simulink library "rlsGradientEst_cl"  (R2018b)
settings: Solver=VariableStepAuto  StartTime=0.0  StopTime=10.0  RelTol=1e-3
undefined symbols (not defined in the file): AdaptationParameter, initBasisParams
libraries: ctrlSharedLib x1
settings Model: Creator=mcobb  LastModifiedBy=mcobb

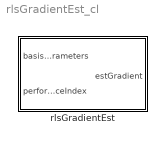
== system rlsGradientEst_cl ==
  rlsGradientEst : Subsystem  mask{InitialParameterData=ones([2*numel(initBasisParams)+1 1]), AdaptationParameter=AdaptationParameter, Ts=1}
      mask prompts: InitialParameterData "Controllib:blocks:recursiveEstimationMaskInitialParameterValues"; AdaptationParameter "Controllib:blocks:recursiveEstimationMaskAdaptationParameterFF"; Ts "Sample Time"
      mask TypeOptions InitialParameterData: Recursive Least Squares Estimator/InitialParameterData
      mask TypeOptions AdaptationParameter: Recursive Least Squares Estimator/AdaptationParameter
      mask DialogControl InitialParameterData Prompt: Initial Parameter Values:
      mask DialogControl AdaptationParameter Prompt: Forgetting Factor:

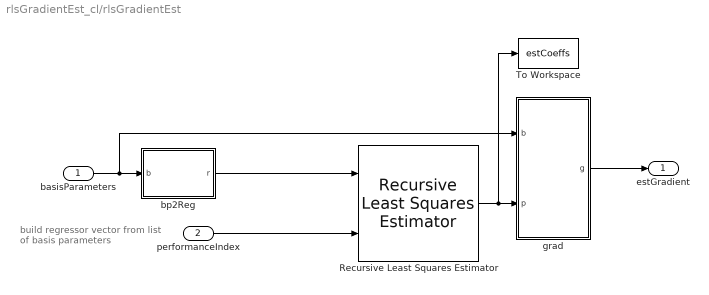
== system rlsGradientEst_cl/rlsGradientEst ==
  note: build regressor vector from
      | list of basis parameters
  basisParameters : Inport
  performanceIndex : Inport  Port=2
  Recursive Least Squares Estimator : ctrlSharedLib/Recursive Least Squares Estimator  InitialEstimateSource=Internal  InitialParameterData=InitialParameterData  P0=1e4  InitialRegressors=0  InitialOutputs=0  History=Infinite  WindowLength=200  EstimationMethod=Forgetting Factor  AdaptationParameter=AdaptationParameter  HasTimeVaryingAdaptationParameter=off  NormalizationBias=eps  OutputError=off  OutputP=off  AddEnablePort=off  InputProcessing=Sample-based  Ts=-1
      settings: SourceProductName=Control System Toolbox  SourceProductBaseCode=CT
  To Workspace : ToWorkspace  VariableName=estCoeffs  SaveFormat=Timeseries  SampleTime=-1
  bp2Reg : MATLAB Function  TreatAsAtomicUnit=on
  grad : MATLAB Function  TreatAsAtomicUnit=on
  estGradient : Outport
  wires:
  bp2Reg/1(r) -> Recursive Least Squares Estimator/1
  performanceIndex/1 -> Recursive Least Squares Estimator/2
  Recursive Least Squares Estimator/1 -> grad/2(p), To Workspace/1
  grad/1(g) -> estGradient/1
  basisParameters/1 -> bp2Reg/1(b), grad/1(b)

== matlab function rlsGradientEst_cl/rlsGradientEst/bp2Reg ==
  data: b input; r output
function r = fcn(b)
% Preallocate column vector output
r = ones(1+2*numel(b),1);
% Build matrix of basis params and their squares
b = [b(:) b(:).^2];
% Reshape to column vector and store into output
r(2:end) = reshape(b',[numel(b),1]);

== matlab function rlsGradientEst_cl/rlsGradientEst/grad ==
  data: b input; g output; p input
function g = fcn(b,p)
p = p(:); % Reshape to column
g = p(2:2:end)+2*p(3:2:end).*b(:);
